simulink model "plant_navigation"  (R2023a)
settings: Solver=VariableStepAuto  StartTime=0.0  StopTime=10.0  RelTol=1e-3
undefined symbols (not defined in the file or in its folder): param
libraries: sharedTrackingLibrary x1, SignalEditorBlockLib x1, aerolibnav x1
settings Model: Creator=timme  LastModifiedBy=timme

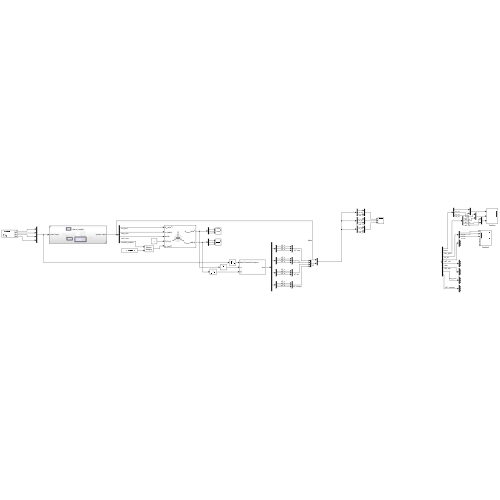
[thumbnail: Simulink's stored preview of the top-level diagram]
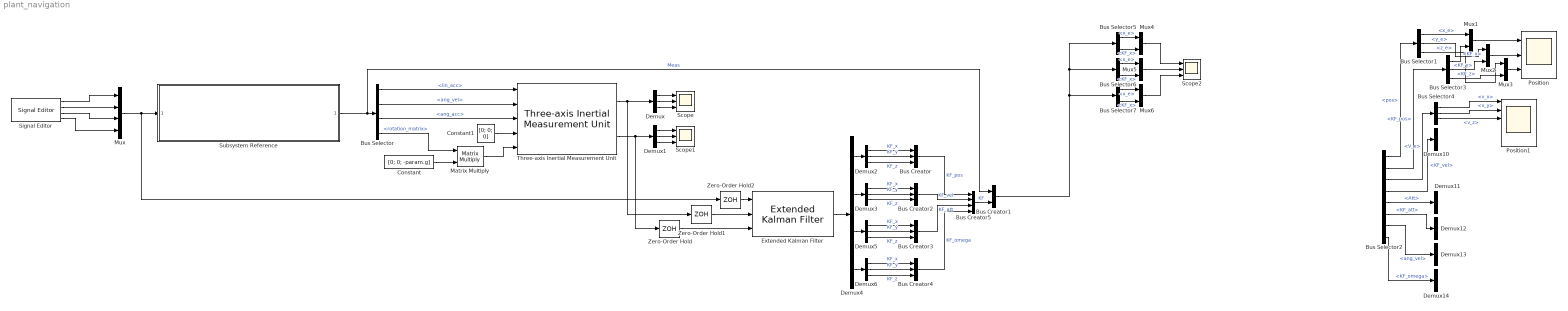
== system plant_navigation ==
  Bus Creator{,2..4} (4 alike) : BusCreator  Inputs=3
  Bus Creator1 : BusCreator  Inputs=2
  Bus Creator5 : BusCreator  Inputs=4
  Bus Selector : BusSelector  OutputSignals=lin_acc,ang_vel,ang_acc,rotation_matrix
  Bus Selector1 : BusSelector  OutputSignals=x_e,y_e,z_e
  Bus Selector2 : BusSelector  OutputSignals=Meas.pos,KF.KF_pos,Meas.V_e,KF.KF_vel,Meas.Att,KF.KF_att,Meas.ang_vel,KF.KF_omega
  Bus Selector3 : BusSelector  OutputSignals=KF_x,KF_y,KF_z
  Bus Selector4 : BusSelector  OutputSignals=v_x,v_y,v_z
  Bus Selector5 : BusSelector  OutputSignals=Meas.pos.x_e,KF.KF_pos.KF_x
  Bus Selector6 : BusSelector  OutputSignals=Meas.pos.x_e,KF.KF_pos.KF_x
  Bus Selector7 : BusSelector  OutputSignals=Meas.pos.x_e,KF.KF_pos.KF_x
  Constant : Constant  Value=[0; 0; -param.g]
  Constant1 : Constant  Value=[0; 0; 0]
  Demux{,1..3,5..6,10..14} (11 alike) : Demux  Outputs=3
  Demux4 : Demux
  Extended Kalman Filter : sharedTrackingLibrary/Extended Kalman Filter  StateTransitionFcn=stateTransition  HasStateTransitionJacobianFcn=off  HasAdditiveProcessNoise=Additive  ProcessNoise=1  HasTimeVaryingProcessNoise=off  HasStateTransitionFcnExtraArgument=1  InitialState=zeros(12,1)  InitialStateCovariance=eye(12)  MeasurementFcn1=accelerometer_model  HasMeasurementJacobianFcn1=off  HasMeasurementEnablePort1=off  HasAdditiveMeasurementNoise1=Additive  MeasurementNoise1=eye(3)  HasTimeVaryingMeasurementNoise1=off  HasMeasurementFcnExtraArgument1=0  HasMeasurementWrapping1=off  MeasurementFcn2=gyrometer_model  HasMeasurementJacobianFcn2=off  HasMeasurementEnablePort2=off  HasAdditiveMeasurementNoise2=Additive  MeasurementNoise2=eye(3)  HasTimeVaryingMeasurementNoise2=off  HasMeasurementFcnExtraArgument2=0  HasMeasurementWrapping2=off  MeasurementFcn3=myMeasurementFcn  HasMeasurementJacobianFcn3=off  HasMeasurementEnablePort3=off  HasAdditiveMeasurementNoise3=Additive  MeasurementNoise3=1  HasTimeVaryingMeasurementNoise3=off  HasMeasurementFcnExtraArgument3=0  HasMeasurementWrapping3=off  MeasurementFcn4=myMeasurementFcn  HasMeasurementJacobianFcn4=off  HasMeasurementEnablePort4=off  HasAdditiveMeasurementNoise4=Additive  MeasurementNoise4=1  HasTimeVaryingMeasurementNoise4=off  HasMeasurementFcnExtraArgument4=0  HasMeasurementWrapping4=off  MeasurementFcn5=myMeasurementFcn  HasMeasurementJacobianFcn5=off  HasMeasurementEnablePort5=off  HasAdditiveMeasurementNoise5=Additive  MeasurementNoise5=1  HasTimeVaryingMeasurementNoise5=off  HasMeasurementFcnExtraArgument5=0  HasMeasurementWrapping5=off  EnableMultirate=off  StateTransitionFcnSampleTime=1  MeasurementFcn1SampleTime=1  MeasurementFcn2SampleTime=1  MeasurementFcn3SampleTime=1  MeasurementFcn4SampleTime=1  MeasurementFcn5SampleTime=1  UseCurrentEstimator=on  OutputStateCovariance=off  DataType=double  SampleTime=0.01  NumberOfMeasurements=2
  Matrix Multiply : Product  Multiplication=Matrix(*)
  Mux : Mux
  Mux{1..6} (6 alike) : Mux  Inputs=2
  Position : Scope  NumInputPorts=3
  Position1 : Scope  NumInputPorts=6
  Scope : Scope  NumInputPorts=3
  Scope1 : Scope  NumInputPorts=3
  Scope2 : Scope  NumInputPorts=3
  Signal Editor : SignalEditorBlockLib/Signal Editor  FileName=C:\Users\timme\OneDrive\Bureaublad\Tu Delft\bsc3\DSE\GNC development\Detailed design phase\navigation\signals\control_inputs.mat  ActiveScenario=Scenario_1  ActiveSignal=T  IsBus=off  OutputBusObjectStr=Bus: BusObject  SampleTime=0  Interpolate=off  ZeroCross=off  OutputAfterFinalValue=Setting to zero  Unit=N  PreserveSignalName=on  ApplySigPropsToAllScenarios=on
  Subsystem Reference : Subsystem  ReferencedSubsystem=drone_model
  Three-axis Inertial Measurement Unit : aerolibnav/Three-axis Inertial Measurement Unit  units=Metric (MKS)  imu=[0 0 0]  i_Ts=0  dtype_a=off  w_a=190  z_a=0.707  a_sf_cc=[1 0 0; 0 1 0; 0 0 1]  a_bias=[0 0 0]  a_sat="[-inf  -inf  -inf  inf inf inf]"  dtype_g=off  w_g=190  z_g=0.707  g_sf_cc=[1 0 0; 0 1 0; 0 0 1]  g_bias=[0 0 0]  g_sens=[0 0 0]  g_sat="[-inf  -inf  -inf  inf inf inf]"  i_rand=on  i_seeds=[23093 23094 23095 23096 23097 23098]  i_pow=[0.00 0.00 0.00 0.000 0.000 0.000]
  Zero-Order Hold : ZeroOrderHold  SampleTime=0.01
  Zero-Order Hold1 : ZeroOrderHold  SampleTime=0.01
  Zero-Order Hold2 : ZeroOrderHold  SampleTime=0.01
  wires:
  Signal Editor/1 -> Mux/1
  Subsystem Reference/1 -> Bus Creator1/1, Bus Selector/1  "Meas"
  Bus Selector/1 -> Three-axis Inertial Measurement Unit/1  "<lin_acc>"
  Bus Selector/2 -> Three-axis Inertial Measurement Unit/2  "<ang_vel>"
  Bus Selector/3 -> Three-axis Inertial Measurement Unit/3  "<ang_acc>"
  Matrix Multiply/1 -> Three-axis Inertial Measurement Unit/5
  Constant/1 -> Matrix Multiply/2
  Bus Selector/4 -> Matrix Multiply/1  "<rotation_matrix>"
  Constant1/1 -> Three-axis Inertial Measurement Unit/4
  Demux/2 -> Scope/2
  Demux/1 -> Scope/1
  Demux/3 -> Scope/3
  Demux1/1 -> Scope1/1
  Demux1/3 -> Scope1/3
  Demux1/2 -> Scope1/2
  Mux/1 -> Zero-Order Hold2/1, Subsystem Reference/1
  Extended Kalman Filter/1 -> Demux4/1
  Three-axis Inertial Measurement Unit/1 -> Zero-Order Hold1/1, Demux/1
  Three-axis Inertial Measurement Unit/2 -> Zero-Order Hold/1, Demux1/1
  Zero-Order Hold/1 -> Extended Kalman Filter/3
  Zero-Order Hold1/1 -> Extended Kalman Filter/2
  Zero-Order Hold2/1 -> Extended Kalman Filter/1
  Signal Editor/2 -> Mux/2
  Signal Editor/3 -> Mux/3
  Signal Editor/4 -> Mux/4
  Demux4/1 -> Demux2/1
  Demux2/1 -> Bus Creator/1  "KF_x"
  Demux2/2 -> Bus Creator/2  "KF_y"
  Demux2/3 -> Bus Creator/3  "KF_z"
  Bus Creator/1 -> Bus Creator5/1  "KF_pos"
  Demux3/1 -> Bus Creator2/1  "KF_x"
  Demux3/2 -> Bus Creator2/2  "KF_y"
  Demux3/3 -> Bus Creator2/3  "KF_z"
  Bus Creator2/1 -> Bus Creator5/2  "KF_vel"
  Demux4/2 -> Demux3/1
  Demux5/1 -> Bus Creator3/1  "KF_x"
  Demux5/2 -> Bus Creator3/2  "KF_y"
  Demux5/3 -> Bus Creator3/3  "KF_z"
  Bus Creator3/1 -> Bus Creator5/3  "KF_att"
  Demux4/3 -> Demux5/1
  Demux6/1 -> Bus Creator4/1  "KF_x"
  Demux6/2 -> Bus Creator4/2  "KF_y"
  Demux6/3 -> Bus Creator4/3  "KF_z"
  Bus Creator4/1 -> Bus Creator5/4  "KF_omega"
  Demux4/4 -> Demux6/1
  Bus Creator5/1 -> Bus Creator1/2  "KF"
  Bus Selector2/1 -> Bus Selector1/1  "<pos>"
  Bus Selector2/2 -> Bus Selector3/1  "<KF_pos>"
  Bus Selector2/3 -> Bus Selector4/1  "<V_e>"
  Bus Selector2/4 -> Demux10/1  "<KF_vel>"
  Bus Selector2/5 -> Demux11/1  "<Att>"
  Bus Selector2/6 -> Demux12/1  "<KF_att>"
  Bus Selector2/7 -> Demux13/1  "<ang_vel>"
  Bus Selector2/8 -> Demux14/1  "<KF_omega>"
  Bus Selector1/1 -> Mux1/1  "<x_e>"
  Bus Selector3/1 -> Mux1/2  "<KF_x>"
  Bus Selector4/1 -> Position1/1  "<v_x>"
  Bus Selector4/2 -> Position1/2  "<v_y>"
  Bus Selector4/3 -> Position1/3  "<v_z>"
  Mux1/1 -> Position/1
  Mux2/1 -> Position/2
  Bus Selector1/2 -> Mux2/1  "<y_e>"
  Bus Selector3/2 -> Mux2/2  "<KF_y>"
  Mux3/1 -> Position/3
  Bus Selector1/3 -> Mux3/1  "<z_e>"
  Bus Selector3/3 -> Mux3/2  "<KF_z>"
  Bus Selector5/1 -> Mux4/1  "<x_e>"
  Bus Selector5/2 -> Mux4/2  "<KF_x>"
  Bus Selector6/1 -> Mux5/1  "<x_e>"
  Bus Selector6/2 -> Mux5/2  "<KF_x>"
  Bus Selector7/2 -> Mux6/2  "<KF_x>"
  Bus Creator1/1 -> Bus Selector7/1, Bus Selector6/1, Bus Selector5/1
  Bus Selector7/1 -> Mux6/1  "<x_e>"
  Mux5/1 -> Scope2/2
  Mux4/1 -> Scope2/1
  Mux6/1 -> Scope2/3
